simulink model "Comp_TestBed_org"  (Simulink 10.0)
settings: Solver=FixedStepDiscrete  StartTime=0.0  StopTime=1  FixedStep=1  RelTol=1e-3  EnableMultiTasking=on
undefined symbols (not defined in the file): MWS
libraries: Lib_Turbo_Compressor_TMATS x1
settings Model: Creator=jwchapm2  LastModifiedBy=annonymous
settings DataIOCC: LimitDataPoints=on
settings OptimizationCC: ExpressionDepthLimit=2147483647
settings DebuggingCC: SolverPrmCheckMsg=warning  StateNameClashWarn=warning
settings GRTTargetCC: GeneratePreprocessorConditionals=Disable all  CombineOutputUpdateFcns=on  GRTInterface=off
settings ConfigComp: CovExternalEMLEnable=off

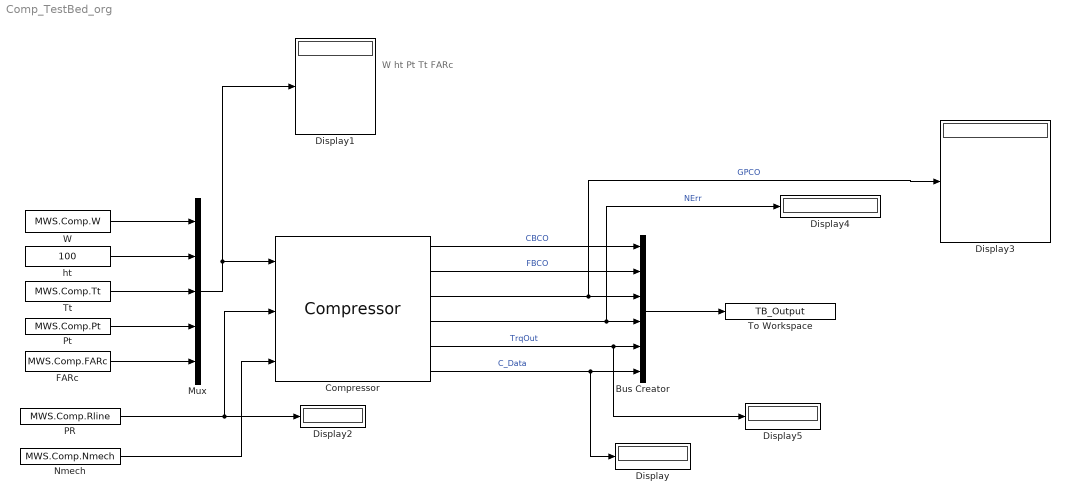
== system Comp_TestBed_org ==
  note: W
      | ht
      | Pt
      | Tt
      | FARc
  Bus Creator : BusCreator  Inputs=6
  Compressor : Lib_Turbo_Compressor_TMATS/Compressor  X_C_RlineVec_M=MWS.Comp.RlineVec  Y_C_NcVec_M=MWS.Comp.NcVec  T_C_Map_WcArray_M=MWS.Comp.WcArray  T_C_Map_PRArray_M=MWS.Comp.PRArray  T_C_Map_EffArray_M=MWS.Comp.EffArray  s_C_Nc_M=MWS.Comp.s_Nc  s_C_Wc_M=MWS.Comp.s_Wc  s_C_PR_M=MWS.Comp.s_PR  s_C_Eff_M=MWS.Comp.s_eff  CBLDEN_M=on  C_CBD_M=MWS.Comp.CBD  C_CBFht_M=MWS.Comp.CBFht  C_CBFPt_M=MWS.Comp.CBFPt  FBLDEN_M=on  C_FBD_M=MWS.Comp.FBD  C_BFht_M=MWS.Comp.FBht  C_BFPt_M=MWS.Comp.FBPt  X_C_WcSurgeVec_M=MWS.Comp.WcSurgeVec  T_C_PRSurgeVec_M=MWS.Comp.PRSugeVec  iDesign_M=off  NcDes_M=10000  EffDes_M=0.95  PRDes_M=20  RlineDes_M=2
  Display{,1..5} (6 alike) : Display
  FARc : Constant  Value=MWS.Comp.FARc
  Mux : Mux  Inputs=5
  Nmech : Constant  Value=MWS.Comp.Nmech
  PR : Constant  Value=MWS.Comp.Rline
  Pt : Constant  Value=MWS.Comp.Pt
  To Workspace : ToWorkspace  VariableName=TB_Output  SampleTime=-1
  Tt : Constant  Value=MWS.Comp.Tt
  W : Constant  Value=MWS.Comp.W
  ht : Constant  Value=100
  wires:
  PR/1 -> Compressor/2, Display2/1
  W/1 -> Mux/1
  FARc/1 -> Mux/5
  Tt/1 -> Mux/3
  Pt/1 -> Mux/4
  Mux/1 -> Compressor/1, Display1/1
  Compressor/3 -> Display3/1, Bus Creator/3  "GPCO"
  Compressor/4 -> Display4/1, Bus Creator/4  "NErr"
  Compressor/5 -> Bus Creator/5, Display5/1  "TrqOut"
  Compressor/6 -> Bus Creator/6, Display/1  "C_Data"
  Bus Creator/1 -> To Workspace/1
  ht/1 -> Mux/2
  Nmech/1 -> Compressor/3
  Compressor/2 -> Bus Creator/2  "FBCO"
  Compressor/1 -> Bus Creator/1  "CBCO"
